simulink model "Compare4Bit"  (R2023a)
settings: Solver=VariableStepAuto  StartTime=0.0  StopTime=1  RelTol=1e-3
settings Model: Creator=Admin  LastModifiedBy=Admin

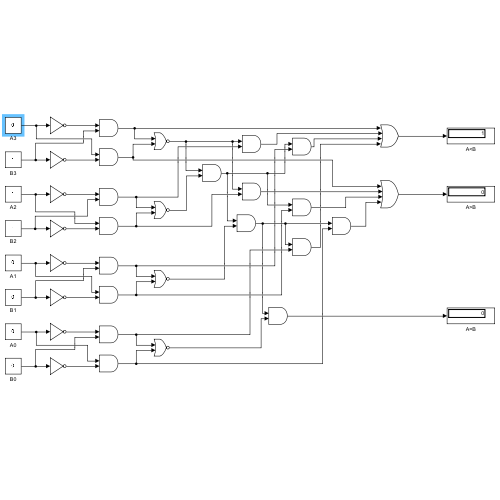
[thumbnail: Simulink's stored preview of the top-level diagram]
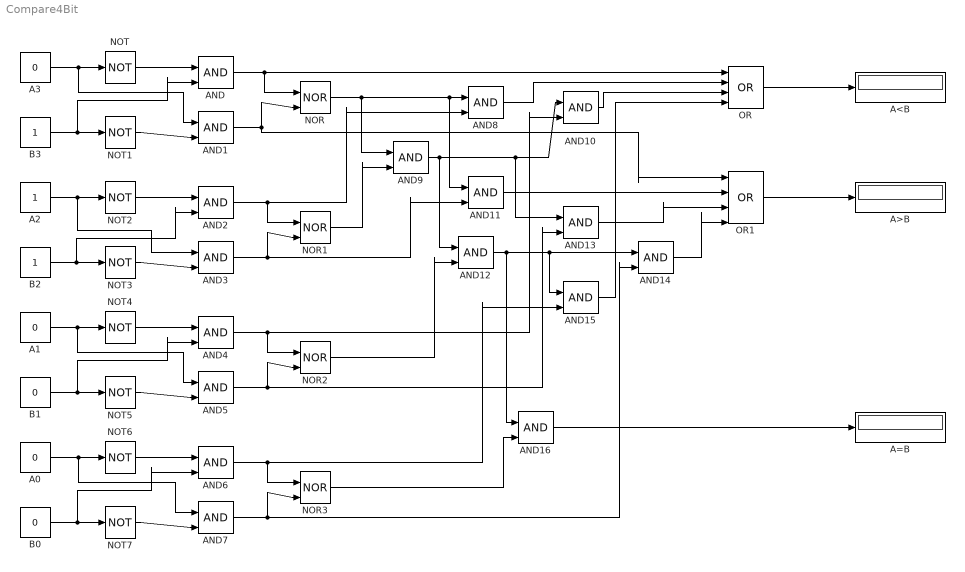
== system Compare4Bit ==
  A0 : Constant  Value=0  SampleTime=-1
  A1 : Constant  Value=0  SampleTime=-1
  A2 : Constant  SampleTime=-1
  A3 : Constant  Value=0  SampleTime=-1
  A<B : Display
  A=B : Display
  A>B : Display
  AND{,1..16} (17 alike) : Logic  IconShape=distinctive  AllPortsSameDT=off  OutDataTypeStr=boolean
  B0 : Constant  Value=0  SampleTime=-1
  B1 : Constant  Value=0  SampleTime=-1
  B2 : Constant  SampleTime=-1
  B3 : Constant  SampleTime=-1
  NOR{,1..3} (4 alike) : Logic  Operator=NOR  IconShape=distinctive  AllPortsSameDT=off  OutDataTypeStr=boolean
  NOT{,1..7} (8 alike) : Logic  Operator=NOT  IconShape=distinctive  AllPortsSameDT=off  OutDataTypeStr=boolean
  OR : Logic  Operator=OR  Inputs=4  IconShape=distinctive  AllPortsSameDT=off  OutDataTypeStr=boolean
  OR1 : Logic  Operator=OR  Inputs=4  IconShape=distinctive  AllPortsSameDT=off  OutDataTypeStr=boolean
  wires:
  A3/1 -> AND1/1, NOT/1
  B3/1 -> AND/2, NOT1/1
  B2/1 -> AND2/2, NOT3/1
  A2/1 -> AND3/1, NOT2/1
  B0/1 -> AND6/2, NOT7/1
  A0/1 -> AND7/1, NOT6/1
  B1/1 -> AND4/2, NOT5/1
  A1/1 -> AND5/1, NOT4/1
  NOT/1 -> AND/1
  NOT1/1 -> AND1/2
  NOT2/1 -> AND2/1
  NOT3/1 -> AND3/2
  NOT4/1 -> AND4/1
  NOT5/1 -> AND5/2
  NOT6/1 -> AND6/1
  NOT7/1 -> AND7/2
  AND/1 -> OR/1, NOR/1
  AND1/1 -> OR1/1, NOR/2
  NOR/1 -> AND9/1, AND11/1, AND8/1
  AND8/1 -> OR/2
  AND2/1 -> AND8/2, NOR1/1
  AND3/1 -> AND11/2, NOR1/2
  AND4/1 -> AND10/2, NOR2/1
  AND5/1 -> AND13/2, NOR2/2
  AND6/1 -> AND15/2, NOR3/1
  AND7/1 -> AND14/2, NOR3/2
  NOR1/1 -> AND9/2
  AND10/1 -> OR/3
  OR/1 -> A<B/1
  AND9/1 -> AND12/1, AND10/1, AND13/1
  NOR2/1 -> AND12/2
  AND11/1 -> OR1/2
  AND13/1 -> OR1/3
  AND12/1 -> AND16/1, AND15/1, AND14/1
  AND14/1 -> OR1/4
  AND15/1 -> OR/4
  NOR3/1 -> AND16/2
  OR1/1 -> A>B/1
  AND16/1 -> A=B/1
